simulink model "simulation"  (R2023b)
settings: Solver=VariableStepAuto  StartTime=0.0  StopTime=8  RelTol=1e-3
undefined symbols (not defined in the file or in its folder): integ_ctrl_tf_z_neg, lead_ctrl1_tf_z_neg, lead_ctrl2_tf_z_neg
libraries: spsTriangleGeneratorLib x2
settings Model: Creator=camil  LastModifiedBy=camil

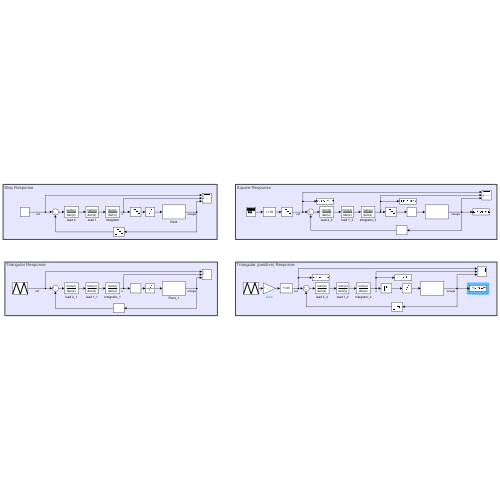
[thumbnail: Simulink's stored preview of the top-level diagram]
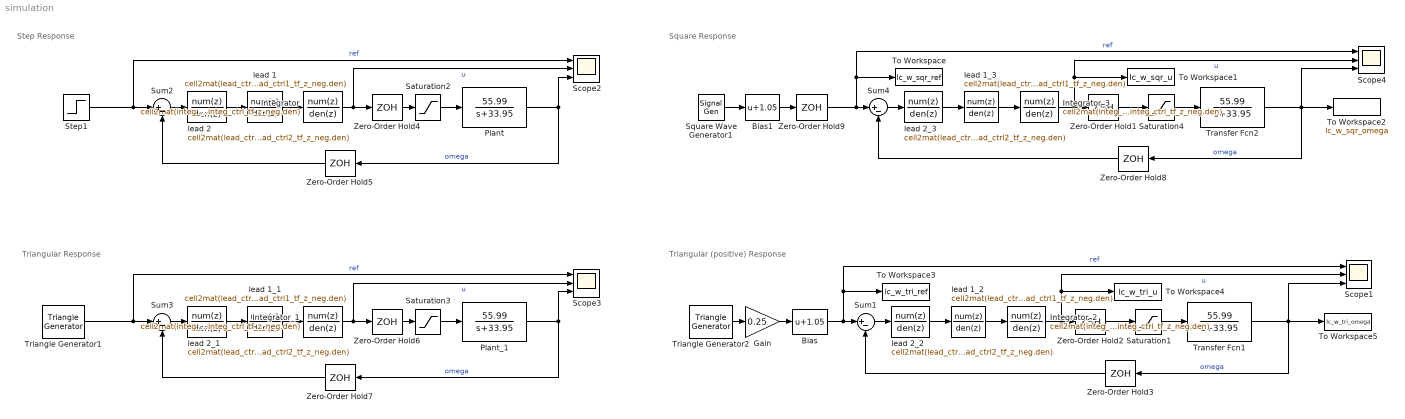
== system simulation ==
  note: Triangular Response
  note: Step Response
  note: Triangular (positive) Response
  note: Square Response
  Bias : Bias  Bias=1.05  SaturateOnIntegerOverflow=off
  Bias1 : Bias  Bias=1.05  SaturateOnIntegerOverflow=off
  Gain : Gain  Gain=0.25
  Integrator : DiscreteFilter  Numerator=cell2mat(integ_ctrl_tf_z_neg.num)  Denominator=cell2mat(integ_ctrl_tf_z_neg.den)
  Integrator_1 : DiscreteFilter  Numerator=cell2mat(integ_ctrl_tf_z_neg.num)  Denominator=cell2mat(integ_ctrl_tf_z_neg.den)
  Integrator_2 : DiscreteFilter  Numerator=cell2mat(integ_ctrl_tf_z_neg.num)  Denominator=cell2mat(integ_ctrl_tf_z_neg.den)
  Integrator_3 : DiscreteFilter  Numerator=cell2mat(integ_ctrl_tf_z_neg.num)  Denominator=cell2mat(integ_ctrl_tf_z_neg.den)
  Plant : TransferFcn  Numerator=[55.99]  Denominator=[1 33.95]
  Plant_1 : TransferFcn  Numerator=[55.99]  Denominator=[1 33.95]
  Saturation{1..4} (4 alike) : Saturate  UpperLimit=1  LowerLimit=-1
  Scope{1..4} (4 alike) : Scope  NumInputPorts=3
  Square Wave Generator1 : SignalGenerator  WaveForm=square  Amplitude=0.25  Frequency=0.25
  Step1 : Step  SampleTime=0.005
  Sum{1..4} (4 alike) : Sum  Inputs=|+-
  To Workspace : ToWorkspace  VariableName=lc_w_sqr_ref  SampleTime=-1
  To Workspace1 : ToWorkspace  VariableName=lc_w_sqr_u  SampleTime=-1
  To Workspace2 : ToWorkspace  VariableName=lc_w_sqr_omega  SampleTime=-1
  To Workspace3 : ToWorkspace  VariableName=lc_w_tri_ref  SampleTime=-1
  To Workspace4 : ToWorkspace  VariableName=lc_w_tri_u  SampleTime=-1
  To Workspace5 : ToWorkspace  VariableName=lc_w_tri_omega  SampleTime=-1
  Transfer Fcn1 : TransferFcn  Numerator=[55.99]  Denominator=[1 33.95]
  Transfer Fcn2 : TransferFcn  Numerator=[55.99]  Denominator=[1 33.95]
  Triangle Generator1 : spsTriangleGeneratorLib/Triangle Generator  Freq=0.25  Phase=0  Ts=0.005
  Triangle Generator2 : spsTriangleGeneratorLib/Triangle Generator  Freq=0.25  Phase=0  Ts=0.005
  Zero-Order Hold{1..9} (9 alike) : ZeroOrderHold  SampleTime=0.005
  lead 1 : DiscreteFilter  Numerator=cell2mat(lead_ctrl1_tf_z_neg.num)  Denominator=cell2mat(lead_ctrl1_tf_z_neg.den)
  lead 1_1 : DiscreteFilter  Numerator=cell2mat(lead_ctrl1_tf_z_neg.num)  Denominator=cell2mat(lead_ctrl1_tf_z_neg.den)
  lead 1_2 : DiscreteFilter  Numerator=cell2mat(lead_ctrl1_tf_z_neg.num)  Denominator=cell2mat(lead_ctrl1_tf_z_neg.den)
  lead 1_3 : DiscreteFilter  Numerator=cell2mat(lead_ctrl1_tf_z_neg.num)  Denominator=cell2mat(lead_ctrl1_tf_z_neg.den)
  lead 2 : DiscreteFilter  Numerator=cell2mat(lead_ctrl2_tf_z_neg.num)  Denominator=cell2mat(lead_ctrl2_tf_z_neg.den)
  lead 2_1 : DiscreteFilter  Numerator=cell2mat(lead_ctrl2_tf_z_neg.num)  Denominator=cell2mat(lead_ctrl2_tf_z_neg.den)
  lead 2_2 : DiscreteFilter  Numerator=cell2mat(lead_ctrl2_tf_z_neg.num)  Denominator=cell2mat(lead_ctrl2_tf_z_neg.den)
  lead 2_3 : DiscreteFilter  Numerator=cell2mat(lead_ctrl2_tf_z_neg.num)  Denominator=cell2mat(lead_ctrl2_tf_z_neg.den)
  wires:
  Zero-Order Hold2/1 -> Saturation1/1
  Integrator_2/1 -> Zero-Order Hold2/1, To Workspace4/1, Scope1/2  "u"
  Zero-Order Hold3/1 -> Sum1/2
  Bias/1 -> Sum1/1, To Workspace3/1, Scope1/1  "ref"
  Sum1/1 -> lead 2_2/1
  Transfer Fcn1/1 -> To Workspace5/1, Scope1/3, Zero-Order Hold3/1  "omega"
  Saturation1/1 -> Transfer Fcn1/1
  Saturation2/1 -> Plant/1
  Zero-Order Hold4/1 -> Saturation2/1
  Step1/1 -> Sum2/1, Scope2/1  "ref"
  Zero-Order Hold5/1 -> Sum2/2
  Plant/1 -> Scope2/3, Zero-Order Hold5/1  "omega"
  Sum2/1 -> lead 2/1
  lead 2/1 -> lead 1/1
  lead 1/1 -> Integrator/1
  Integrator/1 -> Zero-Order Hold4/1, Scope2/2  "u"
  Zero-Order Hold7/1 -> Sum3/2
  lead 1_1/1 -> Integrator_1/1
  Integrator_1/1 -> Zero-Order Hold6/1, Scope3/2  "u"
  Zero-Order Hold6/1 -> Saturation3/1
  lead 2_1/1 -> lead 1_1/1
  Triangle Generator1/1 -> Sum3/1, Scope3/1  "ref"
  Sum3/1 -> lead 2_1/1
  Saturation3/1 -> Plant_1/1
  Plant_1/1 -> Scope3/3, Zero-Order Hold7/1  "omega"
  Triangle Generator2/1 -> Gain/1
  Gain/1 -> Bias/1
  lead 2_2/1 -> lead 1_2/1
  lead 1_2/1 -> Integrator_2/1
  Integrator_3/1 -> Zero-Order Hold1/1, To Workspace1/1, Scope4/2  "u"
  lead 2_3/1 -> lead 1_3/1
  lead 1_3/1 -> Integrator_3/1
  Bias1/1 -> Zero-Order Hold9/1
  Sum4/1 -> lead 2_3/1
  Saturation4/1 -> Transfer Fcn2/1
  Transfer Fcn2/1 -> To Workspace2/1, Scope4/3, Zero-Order Hold8/1  "omega"
  Zero-Order Hold8/1 -> Sum4/2
  Zero-Order Hold1/1 -> Saturation4/1
  Square Wave Generator1/1 -> Bias1/1
  Zero-Order Hold9/1 -> Sum4/1, Scope4/1, To Workspace/1  "ref"
